simulink model "un_tanque_r2018a"  (R2018a)
settings: Solver=ode23tb  StartTime=0.0  StopTime=30.0  RelTol=1e-3  EnableMultiTasking=on
settings Model: Creator=Matias  LastModifiedBy=tomej
settings OptimizationCC: LifeSpan=inf
settings DebuggingCC: SFUnexpectedBacktrackingDiag=warning  SFNoUnconditionalDefaultTransitionDiag=warning  SFExecutionAtInitializationDiag=none
settings CodeAppCC: StateflowObjectComments=on
settings GRTTargetCC: TargetLangStandard=C89/C90 (ANSI)  GeneratePreprocessorConditionals=Disable all
settings ConfigComp: CovMetricSettings=dw  CovHtmlReporting=on  CovSaveCumulativeToWorkspaceVar=on  CovSaveSingleToWorkspaceVar=on  CovExternalEMLEnable=off

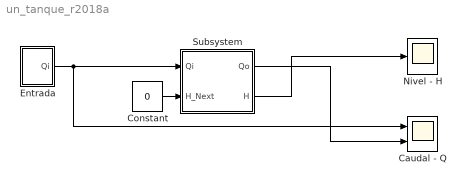
== system un_tanque_r2018a ==
  Caudal - Q : Scope  NumInputPorts=2
  Constant : Constant  Value=0
  Entrada : Subsystem
  Nivel - H : Scope
  Subsystem : Subsystem
  wires:
  Constant/1 -> Subsystem/2(H_Next)
  Entrada/1(Qi) -> Subsystem/1("Qi "), Caudal - Q/1
  Subsystem/1(Qo) -> Caudal - Q/2
  Subsystem/2("H ") -> Nivel - H/1

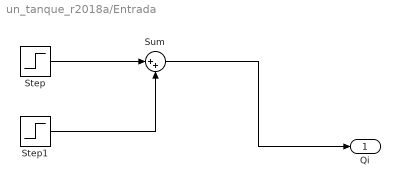
== system un_tanque_r2018a/Entrada ==
  Step : Step  SampleTime=0
  Step1 : Step  Time=15  After=-1  SampleTime=0
  Sum : Sum  Inputs=|++
  Qi : Outport
  wires:
  Step1/1 -> Sum/2
  Step/1 -> Sum/1
  Sum/1 -> Qi/1

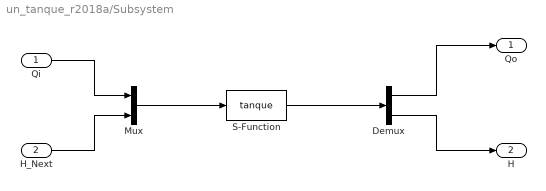
== system un_tanque_r2018a/Subsystem ==
  "Qi " : Inport
  H_Next : Inport  Port=2
  Demux : Demux  Outputs=2
  Mux : Mux  Inputs=2
  S-Function : S-Function  FunctionName=tanque  Parameters=1, 1, 1, 0  SFunctionDeploymentMode=off  EnableBusSupport=off
  Qo : Outport
  "H " : Outport  Port=2
  wires:
  Mux/1 -> S-Function/1
  "Qi "/1 -> Mux/1
  H_Next/1 -> Mux/2
  S-Function/1 -> Demux/1
  Demux/2 -> "H "/1
  Demux/1 -> Qo/1
